simulink model "model2"  (R2022a)
settings: Solver=VariableStepAuto  StartTime=0.0  StopTime=70  RelTol=1e-3
settings Model: Creator=tano-  LastModifiedBy=tano-

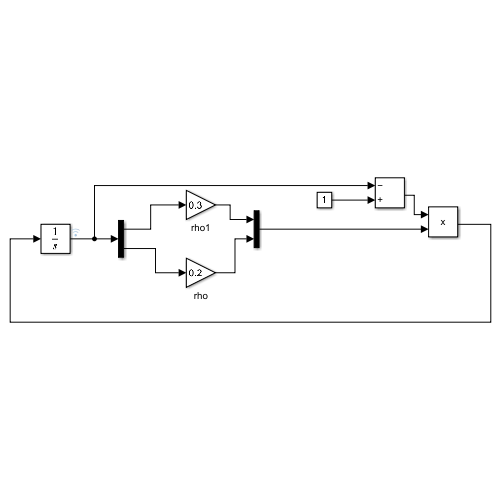
[thumbnail: Simulink's stored preview of the top-level diagram]
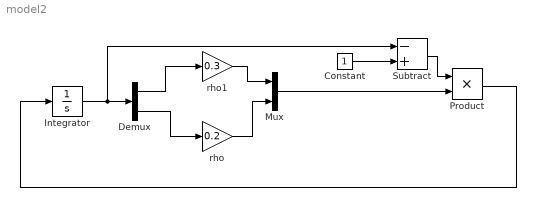
== system model2 ==
  Constant : Constant
  Demux : Demux  Outputs=2
  Integrator : Integrator  InitialCondition=[0.0001 0.0001]
  Mux : Mux  Inputs=2
  Product : Product
  Subtract : Sum  Inputs=-+
  rho : Gain  Gain=0.2
  rho1 : Gain  Gain=0.3
  wires:
  rho1/1 -> Mux/1
  rho/1 -> Mux/2
  Subtract/1 -> Product/1
  Product/1 -> Integrator/1
  Mux/1 -> Product/2
  Constant/1 -> Subtract/2
  Integrator/1 -> Subtract/1, Demux/1
  Demux/1 -> rho1/1
  Demux/2 -> rho/1
